simulink model "controller"  (Simulink 7.0)
settings: Solver=FixedStepDiscrete  StartTime=0.0  StopTime=inf  FixedStep=60  RelTol=1e-3
libraries: simulink x8
settings Model: Creator=mwetter  LastModifiedBy=mwetter  ExtModeAutoUpdateStatusClock=off
settings DebuggingCC: SaveWithParameterizedLinksMsg=none
settings GRTTargetCC: TargetFcnLib=ansi_tfl_tmw.mat

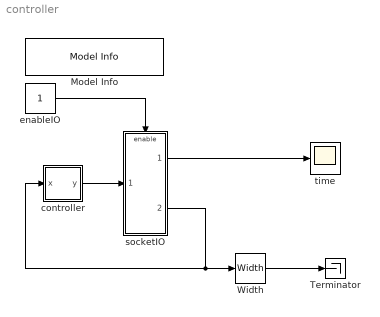
== system controller ==
  Model Info : simulink/Model-Wide Utilities/Model Info  SystemSampleTime=-1  InitialBlockCM=None  BlockCM=None  Frame=off  DisplayStringWithTags=|  HorizontalTextAlignment=Left  LeftAlignmentValue=0.02  SourceBlockDiagram=controller  TagMaxNumber=20
      | Model Info
      | % Set to 1 to enable IO
  Terminator : Terminator
  Width : Width  DataType=int16
  controller : Subsystem
  enableIO : Constant  OutDataType=sfix(16)  OutScaling=2^0
  socketIO : Subsystem
  time : Scope
  wires:
  socketIO/2(dblOut) -> Width/1, controller/1(x)
  socketIO/1(simTim) -> time/1
  Width/1 -> Terminator/1
  enableIO/1 -> socketIO/Enable
  controller/1(y) -> socketIO/1(dblIn)

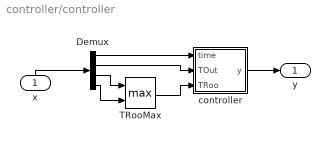
== system controller/controller ==
  x : Inport  Orientation=up
  Demux : Demux
  TRooMax : MinMax  Function=max  Inputs=2  OutDataType=sfix(16)  OutScaling=2^0
  controller : Subsystem
  y : Outport
  wires:
  Demux/1 -> controller/1(time)
  Demux/2 -> controller/2(TOut)
  Demux/3 -> TRooMax/1
  Demux/4 -> TRooMax/2
  TRooMax/1 -> controller/3(TRoo)
  controller/1(y) -> y/1
  x/1 -> Demux/1

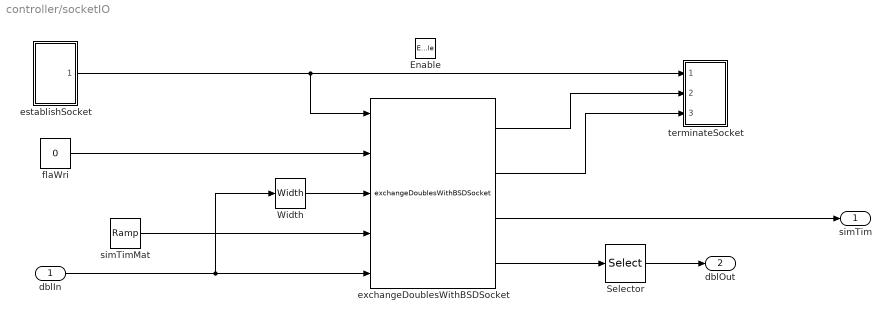
== system controller/socketIO ==
  dblIn : Inport
  Enable : EnablePort
  Selector : Selector  InputPortWidth=128  IndexOptions=Index vector (dialog)  Indices=[1 2 3 4]  OutputSizes=1
  Width : Width  DataType=int16
  establishSocket : Subsystem  TreatAsAtomicUnit=on
  exchangeDoublesWithBSDSocket : S-Function  FunctionName=exchangeDoublesWithBSDSocket  mask(Legacy Function){SFunctionSpec=int16 y1 = exchangeDoublesWithBSDSocket(int16 u1[1], int16 u2[1], int16 y2[1], double u3[1], double u4[], double y3[1], double y4[50]), ShowSpec=off}
      mask prompts: ShowSpec "Display function specification"
      mask help:
      | This block allows the user to call the following C function(s) in Simulink:
      |
      |  InitializeConditionsFcn: none
      |
      |  StartFcn: none
      |
      |  OutputFcn: int16 y1 = exchangeDoublesWithBSDSocket(int16 u1[1], int16 u2[1], int16 y2[1], double u3[1], double u4[], double y3[1], double y4[50])
      |
      |  TerminateFcn: none
      mask CallbackString:
      | |if strcmp(get_param(gcbh, 'ShowSpec'), 'on')
      |   set_param(gcbh, 'MaskDisplay', sprintf('fprintf(''%s'');', get_param(gcbh, 'SFunctionSpec')));
      | else
      |   set_param(gcbh, 'MaskDisplay', sprintf('fprintf(''%s'');', get_param(gcbh, 'FunctionName')));
      | end
      mask Display: fprintf('exchangeDoublesWithBSDSocket');
  flaWri : Constant  Value=0  OutDataTypeMode=int16  OutDataType=sfix(16)  OutScaling=2^0
  simTimMat : simulink/Sources/Ramp  SystemSampleTime=-1  slope=1  start=0  X0=0
  terminateSocket : Subsystem
  simTim : Outport
  dblOut : Outport  Port=2
  wires:
  establishSocket/1(socketFD) -> exchangeDoublesWithBSDSocket/1, terminateSocket/1(sockfd)
  flaWri/1 -> exchangeDoublesWithBSDSocket/2
  exchangeDoublesWithBSDSocket/3 -> simTim/1
  dblIn/1 -> exchangeDoublesWithBSDSocket/5, Width/1
  simTimMat/1 -> exchangeDoublesWithBSDSocket/4
  Width/1 -> exchangeDoublesWithBSDSocket/3
  Selector/1 -> dblOut/1
  exchangeDoublesWithBSDSocket/4 -> Selector/1
  exchangeDoublesWithBSDSocket/1 -> terminateSocket/2(excRetVal)
  exchangeDoublesWithBSDSocket/2 -> terminateSocket/3(excFlaRea)

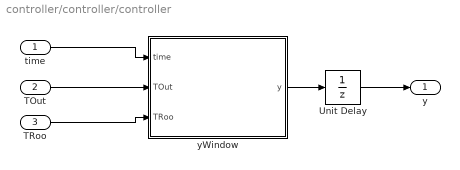
== system controller/controller/controller ==
  time : Inport
  TOut : Inport  Port=2
  TRoo : Inport  Port=3  OutDataType=sfix(16)  OutScaling=2^0
  Unit Delay : UnitDelay  X0=30  SampleTime=-1
  yWindow : Subsystem
  y : Outport
  wires:
  time/1 -> yWindow/1(time)
  TOut/1 -> yWindow/2(TOut)
  Unit Delay/1 -> y/1
  yWindow/1(y) -> Unit Delay/1
  TRoo/1 -> yWindow/3(TRoo)

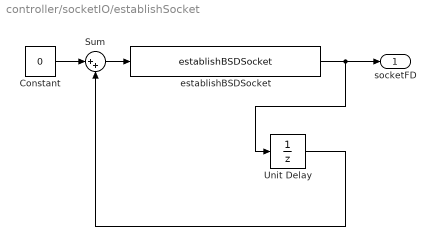
== system controller/socketIO/establishSocket ==
  Constant : Constant  Value=0  OutDataTypeMode=int16  OutDataType=sfix(16)  OutScaling=2^0
  Sum : Sum  Inputs=|++  OutDataType=sfix(16)  OutScaling=2^0
  Unit Delay : UnitDelay  SampleTime=-1
  establishBSDSocket : S-Function  FunctionName=establishBSDSocket  mask(Legacy Function){SFunctionSpec=int16 y1 = establishBSDSocket(void), ShowSpec=on}
      mask prompts: ShowSpec "Display function specification"
      mask help:
      | This block allows the user to call the following C function(s) in Simulink:
      |
      |  InitializeConditionsFcn: none
      |
      |  StartFcn: none
      |
      |  OutputFcn: int16 y1 = establishBSDSocket(void)
      |
      |  TerminateFcn: none
      mask CallbackString:
      | |if strcmp(get_param(gcbh, 'ShowSpec'), 'on')
      |   set_param(gcbh, 'MaskDisplay', sprintf('fprintf(''%s'');', get_param(gcbh, 'SFunctionSpec')));
      | else
      |   set_param(gcbh, 'MaskDisplay', sprintf('fprintf(''%s'');', get_param(gcbh, 'FunctionName')));
      | end
      mask Display: fprintf('int16 y1 = establishBSDSocket(void)');
  socketFD : Outport
  wires:
  establishBSDSocket/1 -> socketFD/1, Unit Delay/1
  Unit Delay/1 -> Sum/2
  Constant/1 -> Sum/1
  Sum/1 -> establishBSDSocket/1

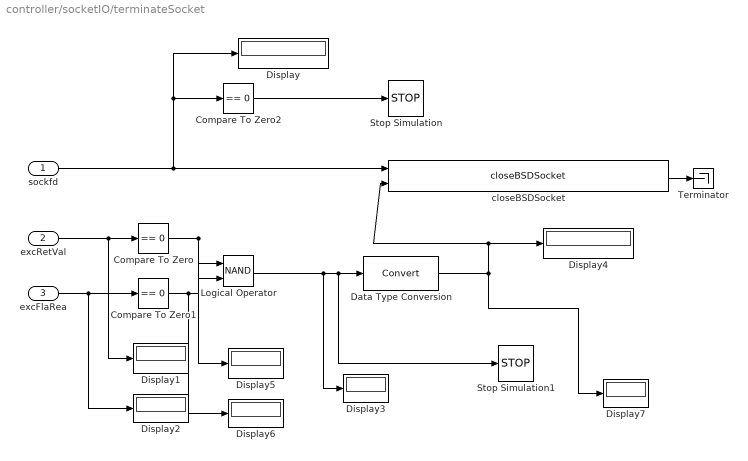
== system controller/socketIO/terminateSocket ==
  sockfd : Inport
  excRetVal : Inport  Port=2
  excFlaRea : Inport  Port=3
  Compare To Zero : simulink/Logic and Bit Operations/Compare To Zero  SystemSampleTime=-1  relop===  LogicOutDataTypeMode=uint8  ZeroCross=off
  Compare To Zero1 : simulink/Logic and Bit Operations/Compare To Zero  SystemSampleTime=-1  relop===  LogicOutDataTypeMode=uint8  ZeroCross=off
  Compare To Zero2 : simulink/Logic and Bit Operations/Compare To Zero  SystemSampleTime=-1  relop===  LogicOutDataTypeMode=boolean  ZeroCross=off
  Data Type Conversion : DataTypeConversion  OutDataType=sfix(16)  OutScaling=2^0
  Display{,1..7} (8 alike) : Display
  Logical Operator : Logic  Operator=NAND  AllPortsSameDT=off  OutDataTypeMode=boolean
  Stop Simulation : Stop
  Stop Simulation1 : Stop
  Terminator : Terminator
  closeBSDSocket : S-Function  FunctionName=closeBSDSocket  mask(Legacy Function){SFunctionSpec=int16 y1 = closeBSDSocket(int16 u1[1], int16 u2[1]), ShowSpec=on}
      mask prompts: ShowSpec "Display function specification"
      mask help:
      | This block allows the user to call the following C function(s) in Simulink:
      |
      |  InitializeConditionsFcn: none
      |
      |  StartFcn: none
      |
      |  OutputFcn: int16 y1 = closeBSDSocket(int16 u1[1], int16 u2[1])
      |
      |  TerminateFcn: none
      mask CallbackString:
      | |if strcmp(get_param(gcbh, 'ShowSpec'), 'on')
      |   set_param(gcbh, 'MaskDisplay', sprintf('fprintf(''%s'');', get_param(gcbh, 'SFunctionSpec')));
      | else
      |   set_param(gcbh, 'MaskDisplay', sprintf('fprintf(''%s'');', get_param(gcbh, 'FunctionName')));
      | end
      mask Display: fprintf('int16 y1 = closeBSDSocket(int16 u1[1], int16 u2[1])');
  wires:
  sockfd/1 -> closeBSDSocket/1, Compare To Zero2/1, Display/1
  excRetVal/1 -> Compare To Zero/1, Display1/1
  excFlaRea/1 -> Compare To Zero1/1, Display2/1
  Compare To Zero/1 -> Logical Operator/1, Display5/1
  Compare To Zero1/1 -> Logical Operator/2, Display6/1
  Logical Operator/1 -> Display3/1, Data Type Conversion/1, Stop Simulation1/1
  Data Type Conversion/1 -> closeBSDSocket/2, Display4/1, Display7/1
  Compare To Zero2/1 -> Stop Simulation/1
  closeBSDSocket/1 -> Terminator/1

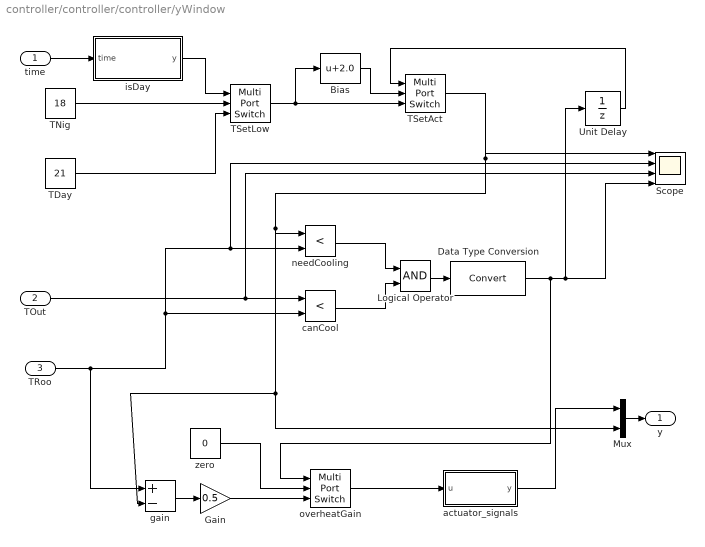
== system controller/controller/controller/yWindow ==
  time : Inport  OutDataType=sfix(16)  OutScaling=2^0
  TOut : Inport  Port=2  OutDataType=sfix(16)  OutScaling=2^0
  TRoo : Inport  Port=3  OutDataType=sfix(16)  OutScaling=2^0
  Bias : Bias  Bias=2.0
  Data Type Conversion : DataTypeConversion  OutDataTypeMode=double  OutDataType=sfix(16)  OutScaling=2^0
  Gain : Gain  Gain=0.5  ParameterDataType=sfix(16)  ParameterScaling=2^0  OutDataType=sfix(16)  OutScaling=2^0
  Logical Operator : Logic  AllPortsSameDT=off  OutDataTypeMode=Specify via dialog  LogicDataType=fixdt(1,16)
  Mux : Mux  Inputs=2
  Scope : Scope  NumInputPorts=4
      settings: TimeRange=600000  YMin=18~17~11~0  YMax=21~26~19~1
  TDay : Constant  Value=21  OutDataType=sfix(16)  OutScaling=2^0
  TNig : Constant  Value=18  OutDataType=sfix(16)  OutScaling=2^0
  TSetAct : MultiPortSwitch  Inputs=2  zeroidx=on  OutDataType=sfix(16)  OutScaling=2^0
  TSetLow : MultiPortSwitch  Inputs=2  zeroidx=on  OutDataType=sfix(16)  OutScaling=2^0
  Unit Delay : UnitDelay  SampleTime=-1
  actuator_signals : Subsystem
  canCool : RelationalOperator  Operator=<  LogicOutDataTypeMode=boolean
  gain : Sum  Inputs=+-  OutDataType=sfix(16)  OutScaling=2^-10
  isDay : Subsystem
  needCooling : RelationalOperator  Operator=<  LogicOutDataTypeMode=boolean
  overheatGain : MultiPortSwitch  Inputs=2  zeroidx=on  OutDataType=sfix(16)  OutScaling=2^0
  zero : Constant  Value=0  OutDataType=sfix(16)  OutScaling=2^0
  y : Outport  OutDataType=sfix(16)  OutScaling=2^0
  wires:
  TOut/1 -> canCool/1, Scope/3
  TDay/1 -> TSetLow/3
  time/1 -> isDay/1(time)
  isDay/1(y) -> TSetLow/1
  TNig/1 -> TSetLow/2
  TRoo/1 -> canCool/2, needCooling/2, Scope/2, gain/1
  needCooling/1 -> Logical Operator/1
  canCool/1 -> Logical Operator/2
  Data Type Conversion/1 -> Unit Delay/1, Scope/4, overheatGain/1
  Mux/1 -> y/1
  Logical Operator/1 -> Data Type Conversion/1
  TSetLow/1 -> TSetAct/3, Bias/1
  Bias/1 -> TSetAct/2
  TSetAct/1 -> needCooling/1, Mux/2, gain/2, Scope/1
  Unit Delay/1 -> TSetAct/1
  gain/1 -> Gain/1
  Gain/1 -> overheatGain/3
  zero/1 -> overheatGain/2
  overheatGain/1 -> actuator_signals/1(u)
  actuator_signals/1(y) -> Mux/1

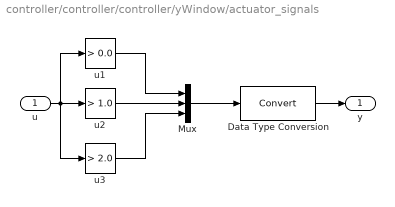
== system controller/controller/controller/yWindow/actuator_signals ==
  u : Inport
  Data Type Conversion : DataTypeConversion  OutDataTypeMode=double  OutDataType=sfix(16)  OutScaling=2^0
  Mux : Mux  Inputs=3
  u1 : simulink/Logic and Bit Operations/Compare To Constant  SystemSampleTime=-1  relop=>  const=0.0  LogicOutDataTypeMode=uint8  ZeroCross=off
  u2 : simulink/Logic and Bit Operations/Compare To Constant  SystemSampleTime=-1  relop=>  const=1.0  LogicOutDataTypeMode=uint8  ZeroCross=off
  u3 : simulink/Logic and Bit Operations/Compare To Constant  SystemSampleTime=-1  relop=>  const=2.0  LogicOutDataTypeMode=uint8  ZeroCross=off
  y : Outport
  wires:
  u/1 -> u1/1, u2/1, u3/1
  u1/1 -> Mux/1
  u2/1 -> Mux/2
  u3/1 -> Mux/3
  Mux/1 -> Data Type Conversion/1
  Data Type Conversion/1 -> y/1

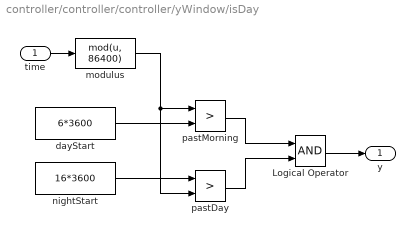
== system controller/controller/controller/yWindow/isDay ==
  time : Inport
  Logical Operator : Logic  AllPortsSameDT=off  OutDataTypeMode=boolean
  dayStart : Constant  Value=6*3600  OutDataType=sfix(16)  OutScaling=2^0
  modulus : MATLABFcn  MATLABFcn=mod(u, 86400)
  nightStart : Constant  Value=16*3600  OutDataType=sfix(16)  OutScaling=2^0
  pastDay : RelationalOperator  Operator=>  LogicOutDataTypeMode=boolean
  pastMorning : RelationalOperator  Operator=>  LogicOutDataTypeMode=boolean
  y : Outport
  wires:
  time/1 -> modulus/1
  modulus/1 -> pastMorning/1, pastDay/2
  dayStart/1 -> pastMorning/2
  nightStart/1 -> pastDay/1
  pastMorning/1 -> Logical Operator/1
  pastDay/1 -> Logical Operator/2
  Logical Operator/1 -> y/1
